simulink model "GateMate_SingleWire_TxRx_RGBW"  (R2025b)
settings: Solver=VariableStepAuto  StartTime=0.0  StopTime=simStopTime  RelTol=1e-3
libraries: ee_lib x17, simulink x9, fl_lib x9, nesl_utility x9
settings Model: Creator=Sneha Shree K  LastModifiedBy=Sneha Shree K

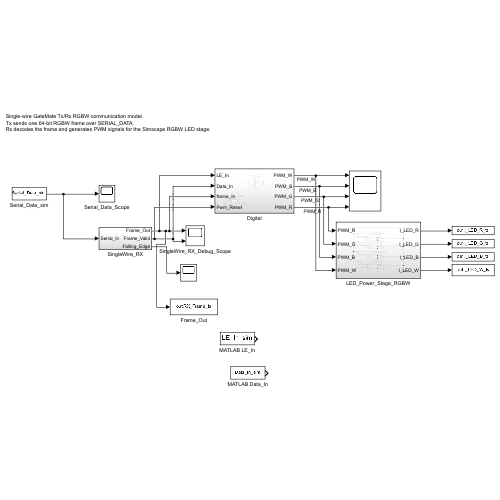
[thumbnail: Simulink's stored preview of the top-level diagram]
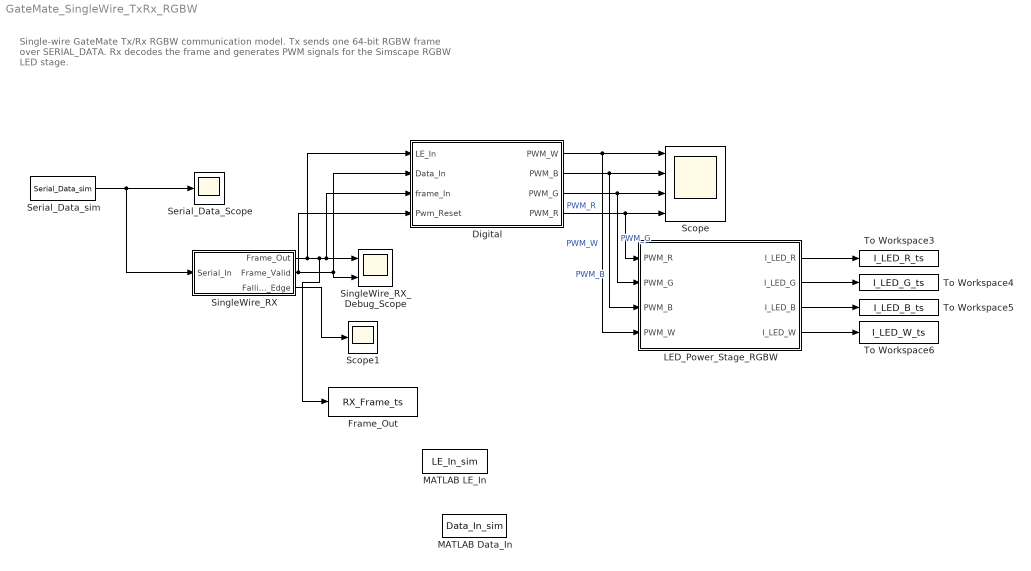
== system GateMate_SingleWire_TxRx_RGBW ==
  note: Single-wire GateMate Tx/Rx RGBW communication model.
      | Tx sends one 64-bit RGBW frame over SERIAL_DATA.
      | Rx decodes the frame and generates PWM signals for the Simscape RGBW LED stage.
  Digital : Subsystem
  Frame_Out : ToWorkspace  VariableName=RX_Frame_ts  SaveFormat=Timeseries  SampleTime=-1
  LED_Power_Stage_RGBW : Subsystem
  MATLAB Data_In : FromWorkspace  VariableName=Data_In_sim  Interpolate=off  OutputAfterFinalValue=Holding final value
  "MATLAB LE_In " : FromWorkspace  VariableName=LE_In_sim  Interpolate=off  OutputAfterFinalValue=Holding final value
  Scope : Scope  NumInputPorts=4
      settings: ActiveDisplayYMinimum=-0.41394567677319716  ActiveDisplayYMaximum=1.1355839256009383
  Scope1 : Scope
      settings: TimeSpan=0.22  ActiveDisplayYMinimum=-0.2  ActiveDisplayYMaximum=1.2  DataLoggingVariableName=ScopeData3
  Serial_Data_Scope : Scope
      settings: ActiveDisplayYMinimum=-0.12499999999999997  ActiveDisplayYMaximum=1.125
  "Serial_Data_sim " : FromWorkspace  VariableName=Serial_Data_sim
  SingleWire_RX : Subsystem
  SingleWire_RX_Debug_Scope : Scope  NumInputPorts=2
      settings: ActiveDisplayYMinimum=-1  ActiveDisplayYMaximum=1  DataLoggingVariableName=ScopeData2
  To Workspace3 : ToWorkspace  VariableName=I_LED_R_ts  SaveFormat=Timeseries  SampleTime=-1
  To Workspace4 : ToWorkspace  VariableName=I_LED_G_ts  SaveFormat=Timeseries  SampleTime=-1
  To Workspace5 : ToWorkspace  VariableName=I_LED_B_ts  SaveFormat=Timeseries  SampleTime=-1
  To Workspace6 : ToWorkspace  VariableName=I_LED_W_ts  SaveFormat=Timeseries  SampleTime=-1
  wires:
  Digital/1(PWM_W) -> LED_Power_Stage_RGBW/4(PWM_W), Scope/1  "PWM_W"
  Digital/2(PWM_B) -> LED_Power_Stage_RGBW/3(PWM_B), Scope/2  "PWM_B"
  Digital/3(PWM_G) -> LED_Power_Stage_RGBW/2(PWM_G), Scope/3  "PWM_G"
  Digital/4(PWM_R) -> LED_Power_Stage_RGBW/1(PWM_R), Scope/4  "PWM_R"
  LED_Power_Stage_RGBW/1(I_LED_R) -> To Workspace3/1
  LED_Power_Stage_RGBW/2(I_LED_G) -> To Workspace4/1
  LED_Power_Stage_RGBW/3(I_LED_B) -> To Workspace5/1
  LED_Power_Stage_RGBW/4(I_LED_W) -> To Workspace6/1
  "Serial_Data_sim "/1 -> SingleWire_RX/1(Serial_In), Serial_Data_Scope/1
  SingleWire_RX/1(Frame_Out) -> Digital/3(frame_In), SingleWire_RX_Debug_Scope/1, Frame_Out/1, Digital/1(LE_In)
  SingleWire_RX/2(Frame_Valid) -> Digital/4(Pwm_Reset), SingleWire_RX_Debug_Scope/2, Digital/2(Data_In)
  SingleWire_RX/3(Falling_Edge) -> Scope1/1

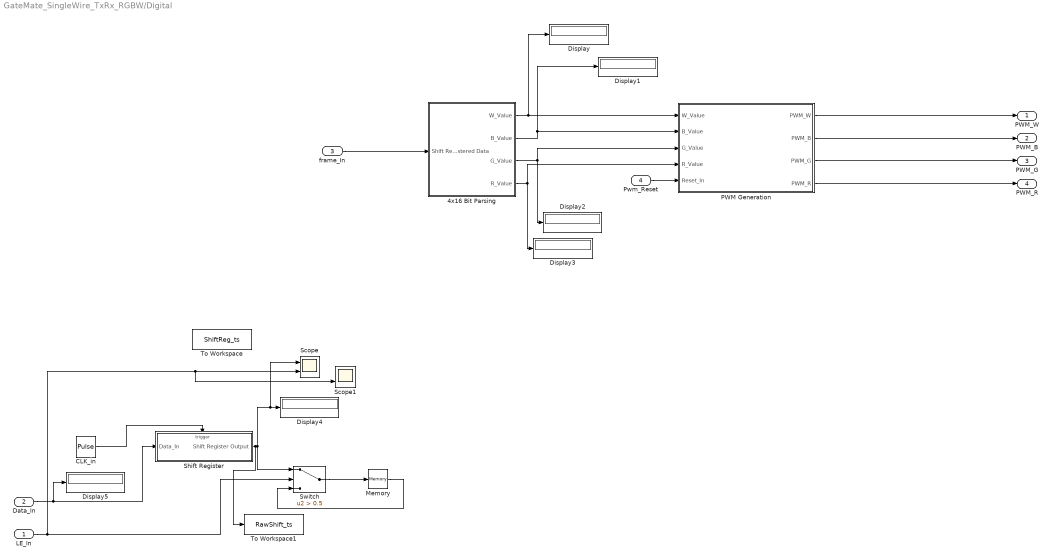
== system GateMate_SingleWire_TxRx_RGBW/Digital ==
  LE_In : Inport
  Data_In : Inport  Port=2
  frame_In : Inport  Port=3  OutDataTypeStr=uint64
  Pwm_Reset : Inport  Port=4  OutDataTypeStr=boolean
  4x16 Bit Parsing : Subsystem
  CLK_in : DiscretePulseGenerator  PulseType=Time based  Period=1e-3  PulseWidth=50  PhaseDelay=0.5e-3
  Display{,1..5} (6 alike) : Display
  Memory : Memory
  PWM Generation : Subsystem
  Scope : Scope  NumInputPorts=2
      settings: ActiveDisplayYMinimum=-0.12499999999999997  ActiveDisplayYMaximum=1.125  DataLoggingVariableName=ScopeData4
  Scope1 : Scope  NumInputPorts=2
      settings: ActiveDisplayYMinimum=-0.12499999999999997  ActiveDisplayYMaximum=1.125  DataLoggingVariableName=ScopeData5
  Shift Register : Subsystem  TreatAsAtomicUnit=on
  Switch : Switch  Criteria=u2 > Threshold  Threshold=0.5  SaturateOnIntegerOverflow=off  InputSameDT=off
  To Workspace : ToWorkspace  VariableName=ShiftReg_ts  SaveFormat=Timeseries  SampleTime=-1
  To Workspace1 : ToWorkspace  VariableName=RawShift_ts  SaveFormat=Timeseries  SampleTime=-1
  PWM_W : Outport
  PWM_B : Outport  Port=2
  PWM_G : Outport  Port=3
  PWM_R : Outport  Port=4
  wires:
  CLK_in/1 -> Shift Register/Trigger
  Data_In/1 -> Display5/1, Shift Register/1(Data_In)
  Switch/1 -> Memory/1
  Memory/1 -> Switch/3
  Shift Register/1(Shift Register Output) -> To Workspace1/1, Scope/1, Display4/1, Switch/1
  LE_In/1 -> Scope1/2, Scope/2, Switch/2
  4x16 Bit Parsing/1(W_Value) -> Display/1, PWM Generation/1(W_Value)
  4x16 Bit Parsing/2(B_Value) -> Display1/1, PWM Generation/2(B_Value)
  4x16 Bit Parsing/3(G_Value) -> Display2/1, PWM Generation/3(G_Value)
  4x16 Bit Parsing/4(R_Value) -> Display3/1, PWM Generation/4(R_Value)
  PWM Generation/1(PWM_W) -> PWM_W/1
  PWM Generation/2(PWM_B) -> PWM_B/1
  PWM Generation/3(PWM_G) -> PWM_G/1
  PWM Generation/4(PWM_R) -> PWM_R/1
  frame_In/1 -> 4x16 Bit Parsing/1(Shift Registered Data)
  Pwm_Reset/1 -> PWM Generation/5(Reset_In)

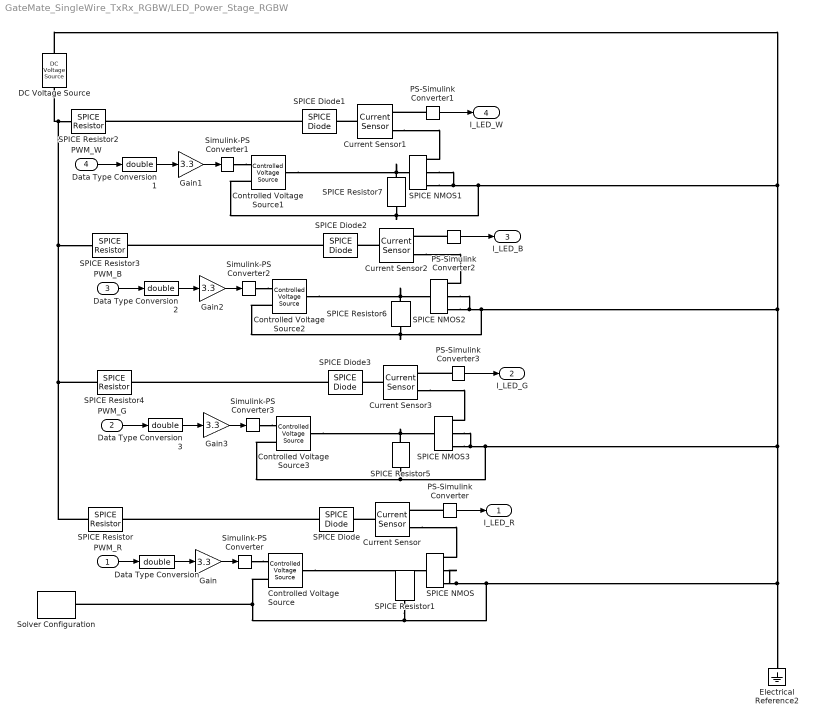
== system GateMate_SingleWire_TxRx_RGBW/LED_Power_Stage_RGBW ==
  PWM_R : Inport
  PWM_G : Inport  Port=2
  PWM_B : Inport  Port=3
  PWM_W : Inport  Port=4
  Controlled Voltage Source{,1..3} (4 alike) : fl_lib/Electrical/Electrical Sources/Controlled Voltage Source
  Current Sensor{,1..3} (4 alike) : fl_lib/Electrical/Electrical Sensors/Current Sensor
  DC Voltage Source : ee_lib/Additional Components/SPICE Sources/DC Voltage Source  DC=12 V
  Data Type Conversion{,1..3} (4 alike) : DataTypeConversion  OutDataTypeStr=double  SaturateOnIntegerOverflow=off  RndMeth=Floor
  Electrical Reference2 : fl_lib/Electrical/Electrical Elements/Electrical Reference
  Gain{,1..3} (4 alike) : Gain  Gain=3.3
  PS-Simulink Converter{,1..3} (4 alike) : nesl_utility/PS-Simulink Converter  PhysicalDomain=network_engine_domain  SubClassName=ps_output  LeftPortType=input  RightPortType=output  PseudoPeriodic=off  Frequencies=[]  VectorFormat=inherit  Unit=A  AffineConversion=off
  SPICE Diode{,1..3} (4 alike) : ee_lib/Additional Components/SPICE Semiconductors/SPICE Diode  AREA=1.0 m^2  SCALE=1  IS=1e-14 A/m^2  IKF=Inf A/m^2  ISR=0 A/m^2  N=1  NR=2  M=0.5  VJ=1 V  RS=0.01 Ohm*m^2  C_param=1  CJO=0 F/m^2  FC=0.5  TT=0 s  IC_given=1  V0=0 V  RevBrk=1  BV=Inf V  IBV=1e-10 A/m^2  IBVL=0 A/m^2  NBV=1  NBVL=1  T_param=1  XTI=3.0  EG=1.11 eV  TIKF=0 1/K  TRS1=0 1/K  TRS2=0 1/K^2  TBV1=0 1/K  TBV2=0 1/K^2  TFIXED=300.15 K  TMEAS=300.15 K  TOFFSET=0 K
      settings: InternalSimscapePortConfiguration="{\"Bottom\":[],\"Left\":[{\"id\":\"p\",\"label\":\"+\",\"type\":\"foundation.electrical.electrical\"}],\"Right\":[{\"id\":\"n\",\"label\":\"-\",\"type\":\"foundation.electrical.electrical\"}],\"Top\":[]}"
  SPICE NMOS{,1..3} (4 alike) : ee_lib/Additional Components/SPICE Semiconductors/SPICE NMOS  LEVEL=1  AREA=1.0  SCALE=1  LENGTH=1e-4 m  WIDTH=1e-4 m  AD=0 m^2  AS=0 m^2  PD=0 m  PS=0 m  NRD=0  NRS=0  RD=0.05 Ohm  RS=0.05 Ohm  RSH=0 Ohm  VTO=1.5 V  KP=1 A/V^2  GAMMA=0 V^(1/2)  PHI=0.6 V  LAMBDA=0 1/V  IS=1e-14 A  N=1  JS=0 A/m^2  DELTA=0  VMAX=0 m/s  NFS=0 1/cm^2  ETA=0  THETA=0 1/V  KAPPA=0.2  Ci_param=ee.enum.intrinsicCapacitance.none  Cov_param=ee.enum.includeCapacitance.no  CGSO=0 F/m  CGDO=0 F/m  CGBO=0 F/m  C_param=ee.enum.includeCapacitance.no  CBD=0 F  CBS=0 F  PB=0.8 V  CJ=0 F/m^2  MJ=0.5  CJSW=0 F/m  MJSW=0.5  FC=0.5  IC_given=ee.enum.initialCondition.no  ICVDS=0 V  ICVGS=0 V  ICVBS=0 V  TOX=1e-7 m  LD=0 m  U0=600 cm^2/(V*s)  NSUB=NaN 1/cm^3  TPG=1  NSS=NaN 1/cm^2  XJ=0 m  T_param=1  TFIXED=300.15 K  TMEAS=300.15 K  TOFFSET=0 K  UEXP=0  UCRIT=1e4 V/cm  NEFF=1  MTYPE=1
      settings: InternalSimscapePortConfiguration="{\"Bottom\":[],\"Left\":[{\"id\":\"gx\",\"label\":\"\",\"type\":\"foundation.electrical.electrical\"}],\"Right\":[{\"id\":\"dx\",\"label\":\"\",\"type\":\"foundation.electrical.electrical\"},{\"id\":\"bx\",\"label\":\"\",\"type\":\"foundation.electrical.electrical\"},{\"id\":\"sx\",\"label\":\"\",\"type\":\"foundation.electrical.electrical\"}],\"Top\":[]}"
  SPICE Resistor{,2..4} (4 alike) : ee_lib/Additional Components/SPICE Passives/SPICE Resistor  SCALE=1.0  R_param=1  R=510 Ohm  RSH=0 Ohm  LENGTH=1e-6 m  WIDTH=1e-6 m  NARROW=0 m  T_param=1  TC1=0 1/K  TC2=0 1/K^2  TOFFSET=0 K  TFIXED=300.15 K  TMEAS=300.15 K
      settings: InternalSimscapePortConfiguration="{\"Bottom\":[],\"Left\":[{\"id\":\"p\",\"label\":\"\",\"type\":\"foundation.electrical.electrical\"}],\"Right\":[{\"id\":\"n\",\"label\":\"\",\"type\":\"foundation.electrical.electrical\"}],\"Top\":[]}"
  SPICE Resistor{1,5..7} (4 alike) : ee_lib/Additional Components/SPICE Passives/SPICE Resistor  SCALE=1.0  R_param=1  R=100 kOhm  RSH=0 Ohm  LENGTH=1e-6 m  WIDTH=1e-6 m  NARROW=0 m  T_param=1  TC1=0 1/K  TC2=0 1/K^2  TOFFSET=0 K  TFIXED=300.15 K  TMEAS=300.15 K
      settings: InternalSimscapePortConfiguration="{\"Bottom\":[],\"Left\":[{\"id\":\"p\",\"label\":\"\",\"type\":\"foundation.electrical.electrical\"}],\"Right\":[{\"id\":\"n\",\"label\":\"\",\"type\":\"foundation.electrical.electrical\"}],\"Top\":[]}"
  Simulink-PS Converter{,1..3} (4 alike) : nesl_utility/Simulink-PS Converter  PhysicalDomain=network_engine_domain  SubClassName=ps_input  LeftPortType=input  RightPortType=output  PseudoPeriodic=off  Frequencies=[]  NoiseDistribution=none  NoiseParameters=[]  Unit=V  AffineConversion=off  FilteringAndDerivatives=provide  SimscapeFilterOrder=1  InputFilterTimeConstant=0.001  UdotUserProvided=0
  Solver Configuration : nesl_utility/Solver Configuration  PhysicalDomain=network_engine_domain  SubClassName=solver  LeftPortType=input  RightPortType=generic  Tones=[]  Harmonics=[]  SimulateNoise=off  Profile=off  UseLocalSampling=off  EnableSwitchedLinearOptims=on  FrequencyDomain=off  UseCCode=off  RelTol=0.001  AbsTol=0.001  MinStep=1e-09  ToWorkspace=off  RevertToSquareIcSolve=off  NumHomotopyIterations=100  PhasorMode=off  PhasorModeNumHarmonics=1  ConsistencySolver=NEWTON_XTOL_AFTER_FTOL  IndexReductionMethod=DerivativeReplacement  DoDC=off  ResidualTolerance=1e-09  ConsistencyTolSource=GLOBAL  ConsistencyAbsTol=0.001  ConsistencyRelTol=0.001  ConsistencyTolFactor=0.001  UseLocalSolver=off  LocalSolverChoice=NE_BACKWARD_EULER_ADVANCER  ResolveIndetEquations=on  FunctionEvalNumThread=1  LocalSolverSampleTime=0.001  DoFixedCost=off  MaxNonlinIter=3  MaxModeIter=2  ComputeImpulses=off  ImpulseIterations=2  LinearAlgebra=auto  LinearAlgebraNumThread=0  EquationFormulation=NE_TIME_EF  DelaysMemoryBudget=1024  AutomaticFiltering=on  FilteringTimeConstant=0.001  PartitionStorageMethod=AS_NEEDED  PartitionMemoryBudget=1024  PartitionMethod=ROBUST  MultibodyUseLocalSolver=off  MultibodyLocalSolverChoice=ODE1  MultibodyLocalSolverSampleTime=0.001
  I_LED_R : Outport  VectorParamsAs1DForOutWhenUnconnected=off
  I_LED_G : Outport  Port=2  VectorParamsAs1DForOutWhenUnconnected=off
  I_LED_B : Outport  Port=3  VectorParamsAs1DForOutWhenUnconnected=off
  I_LED_W : Outport  Port=4  VectorParamsAs1DForOutWhenUnconnected=off
  wires:
  Gain/1 -> Simulink-PS Converter/1
  PS-Simulink Converter/1 -> I_LED_R/1
  PWM_R/1 -> Data Type Conversion/1
  Data Type Conversion/1 -> Gain/1
  Data Type Conversion1/1 -> Gain1/1
  Gain1/1 -> Simulink-PS Converter1/1
  PWM_W/1 -> Data Type Conversion1/1
  PS-Simulink Converter1/1 -> I_LED_W/1
  Data Type Conversion2/1 -> Gain2/1
  Gain2/1 -> Simulink-PS Converter2/1
  PWM_B/1 -> Data Type Conversion2/1
  PS-Simulink Converter2/1 -> I_LED_B/1
  Data Type Conversion3/1 -> Gain3/1
  Gain3/1 -> Simulink-PS Converter3/1
  PWM_G/1 -> Data Type Conversion3/1
  PS-Simulink Converter3/1 -> I_LED_G/1
  connections:
  SPICE Diode/LConn1 -- SPICE Resistor/RConn1
  Current Sensor/LConn1 -- SPICE Diode/RConn1
  Current Sensor/RConn2 -- SPICE NMOS/RConn1
  Controlled Voltage Source/LConn1 -- SPICE NMOS/LConn1
  Simulink-PS Converter/RConn1 -- Controlled Voltage Source/RConn1
  PS-Simulink Converter/LConn1 -- Current Sensor/RConn1
  SPICE Diode1/LConn1 -- SPICE Resistor2/RConn1
  Controlled Voltage Source1/LConn1 -- SPICE Resistor7/LConn1 -- SPICE NMOS1/LConn1
  Current Sensor1/RConn2 -- SPICE NMOS1/RConn1
  PS-Simulink Converter1/LConn1 -- Current Sensor1/RConn1
  Current Sensor1/LConn1 -- SPICE Diode1/RConn1
  Simulink-PS Converter1/RConn1 -- Controlled Voltage Source1/RConn1
  SPICE Diode2/LConn1 -- SPICE Resistor3/RConn1
  Controlled Voltage Source2/LConn1 -- SPICE Resistor6/LConn1 -- SPICE NMOS2/LConn1
  Current Sensor2/RConn2 -- SPICE NMOS2/RConn1
  PS-Simulink Converter2/LConn1 -- Current Sensor2/RConn1
  Current Sensor2/LConn1 -- SPICE Diode2/RConn1
  Simulink-PS Converter2/RConn1 -- Controlled Voltage Source2/RConn1
  SPICE Resistor/LConn1 -- SPICE Resistor4/LConn1 -- SPICE Resistor3/LConn1 -- DC Voltage Source/LConn1 -- SPICE Resistor2/LConn1
  SPICE Diode3/LConn1 -- SPICE Resistor4/RConn1
  Controlled Voltage Source3/LConn1 -- SPICE Resistor5/LConn1 -- SPICE NMOS3/LConn1
  Current Sensor3/RConn2 -- SPICE NMOS3/RConn1
  PS-Simulink Converter3/LConn1 -- Current Sensor3/RConn1
  Current Sensor3/LConn1 -- SPICE Diode3/RConn1
  Simulink-PS Converter3/RConn1 -- Controlled Voltage Source3/RConn1
  Controlled Voltage Source/RConn2 -- SPICE NMOS/RConn2 -- SPICE NMOS/RConn3 -- SPICE Resistor5/RConn1 -- Controlled Voltage Source3/RConn2 -- SPICE NMOS3/RConn2 -- SPICE NMOS3/RConn3 -- SPICE Resistor7/RConn1 -- Controlled Voltage Source1/RConn2 -- SPICE NMOS1/RConn2 -- SPICE NMOS1/RConn3 -- DC Voltage Source/RConn1 -- SPICE Resistor6/RConn1 -- Controlled Voltage Source2/RConn2 -- SPICE NMOS2/RConn2 -- SPICE NMOS2/RConn3 -- Electrical Reference2/LConn1 -- SPICE Resistor1/RConn1 -- Solver Configuration/RConn1

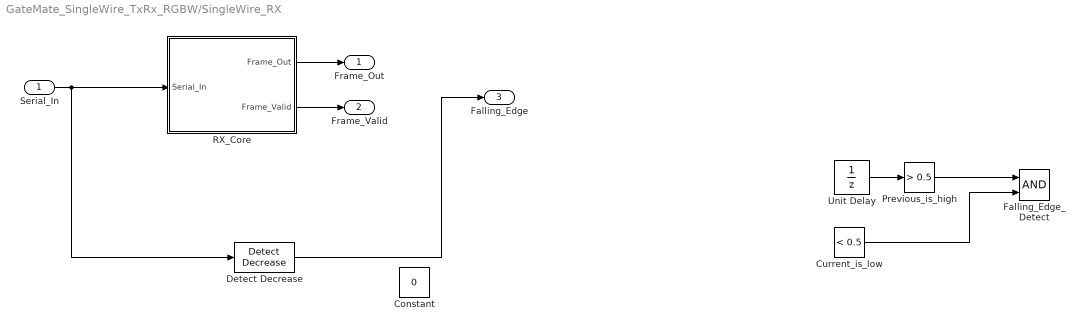
== system GateMate_SingleWire_TxRx_RGBW/SingleWire_RX ==
  Serial_In : Inport
  Constant : Constant  Value=0
  Current_is_low : simulink/Logic and Bit Operations/Compare To Constant  relop=<  const=0.5  OutDataTypeStr=boolean
  Detect Decrease : simulink/Logic and Bit Operations/Detect Decrease  vinit=0.0  OutDataTypeStr=boolean
  Falling_Edge_Detect : Logic  AllPortsSameDT=off  OutDataTypeStr=boolean
  Previous_is_high : simulink/Logic and Bit Operations/Compare To Constant  relop=>  const=0.5  OutDataTypeStr=boolean
  RX_Core : MATLAB Function  TreatAsAtomicUnit=on
  Unit Delay : UnitDelay  InitialCondition=1  HasFrameUpgradeWarning=on
  Frame_Out : Outport  OutDataTypeStr=uint64
  Frame_Valid : Outport  Port=2  OutDataTypeStr=boolean
  Falling_Edge : Outport  Port=3
  wires:
  Serial_In/1 -> RX_Core/1(Serial_In), Detect Decrease/1
  Detect Decrease/1 -> Falling_Edge/1
  ? -> Current_is_low/1, Unit Delay/1
  Unit Delay/1 -> Previous_is_high/1
  Previous_is_high/1 -> Falling_Edge_Detect/1
  Current_is_low/1 -> Falling_Edge_Detect/2
  RX_Core/1(Frame_Out) -> Frame_Out/1
  RX_Core/2(Frame_Valid) -> Frame_Valid/1

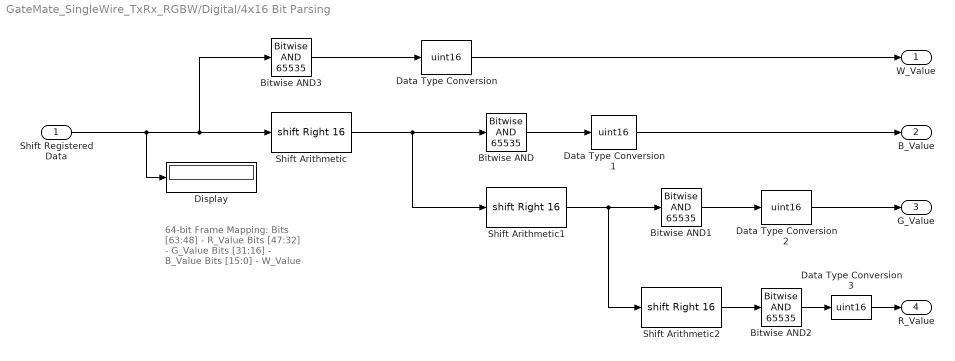
== system GateMate_SingleWire_TxRx_RGBW/Digital/4x16 Bit Parsing ==
  note: 64-bit Frame Mapping:
      |
      | Bits [63:48] - R_Value
      | Bits [47:32] - G_Value
      | Bits [31:16] - B_Value
      | Bits [15:0] - W_Value
  Shift Registered Data : Inport  OutDataTypeStr=uint64
  Bitwise AND{,1..3} (4 alike) : simulink/Logic and Bit Operations/Bitwise Operator  logicop=AND  UseBitMask=on  BitMask=65535  BitMaskRealWorld=Stored Integer
      settings: LibrarySourceBlock=|
      | simulink/Quick Insert/Logic and Bit
      | Operations/Bitwise AND
  Data Type Conversion{,1..3} (4 alike) : DataTypeConversion  OutDataTypeStr=uint16  SaturateOnIntegerOverflow=off  RndMeth=Floor
  Display : Display
  Shift Arithmetic : ArithShift  BitShiftNumber=16  BitShiftDirection=Right
  Shift Arithmetic1 : ArithShift  BitShiftNumber=16  BitShiftDirection=Right
  Shift Arithmetic2 : ArithShift  BitShiftNumber=16  BitShiftDirection=Right
  W_Value : Outport
  B_Value : Outport  Port=2
  G_Value : Outport  Port=3
  R_Value : Outport  Port=4
  wires:
  Shift Arithmetic/1 -> Shift Arithmetic1/1, Bitwise AND/1
  Shift Registered Data/1 -> Display/1, Shift Arithmetic/1, Bitwise AND3/1
  Shift Arithmetic1/1 -> Shift Arithmetic2/1, Bitwise AND1/1
  Shift Arithmetic2/1 -> Bitwise AND2/1
  Bitwise AND3/1 -> Data Type Conversion/1
  Bitwise AND/1 -> Data Type Conversion1/1
  Bitwise AND1/1 -> Data Type Conversion2/1
  Bitwise AND2/1 -> Data Type Conversion3/1
  Data Type Conversion/1 -> W_Value/1
  Data Type Conversion1/1 -> B_Value/1
  Data Type Conversion2/1 -> G_Value/1
  Data Type Conversion3/1 -> R_Value/1

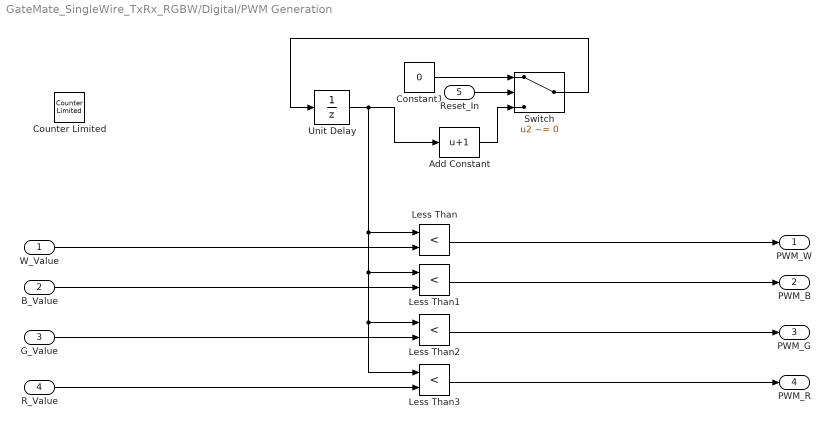
== system GateMate_SingleWire_TxRx_RGBW/Digital/PWM Generation ==
  W_Value : Inport
  B_Value : Inport  Port=2
  G_Value : Inport  Port=3
  R_Value : Inport  Port=4
  Reset_In : Inport  Port=5
  Add Constant : Bias  Bias=1  SaturateOnIntegerOverflow=off
  Constant1 : Constant  Value=0  OutDataTypeStr=uint16
  Counter Limited : simulink/Sources/Counter Limited  uplimit=65535  tsamp=1e-6
  Less Than{,1..3} (4 alike) : RelationalOperator  Operator=<  OutDataTypeStr=boolean  RndMeth=Simplest  InputSameDT=off
  Switch : Switch  Criteria=u2 ~= 0  SaturateOnIntegerOverflow=off  InputSameDT=off
  Unit Delay : UnitDelay  SampleTime=1e-6  HasFrameUpgradeWarning=on
  PWM_W : Outport
  PWM_B : Outport  Port=2
  PWM_G : Outport  Port=3
  PWM_R : Outport  Port=4
  wires:
  W_Value/1 -> Less Than/2
  Less Than/1 -> PWM_W/1
  B_Value/1 -> Less Than1/2
  G_Value/1 -> Less Than2/2
  Less Than1/1 -> PWM_B/1
  Less Than2/1 -> PWM_G/1
  Less Than3/1 -> PWM_R/1
  R_Value/1 -> Less Than3/2
  Constant1/1 -> Switch/1
  Reset_In/1 -> Switch/2
  Add Constant/1 -> Switch/3
  Unit Delay/1 -> Less Than2/1, Less Than3/1, Less Than1/1, Less Than/1, Add Constant/1
  Switch/1 -> Unit Delay/1

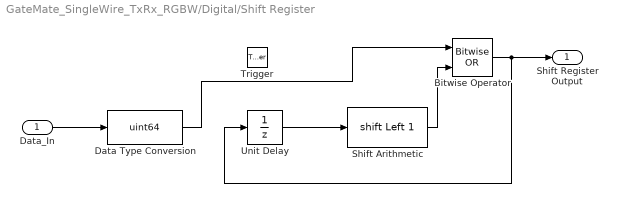
== system GateMate_SingleWire_TxRx_RGBW/Digital/Shift Register ==
  Data_In : Inport
  Trigger : TriggerPort  VariantControl=(inherit)
  Bitwise Operator : simulink/Logic and Bit Operations/Bitwise Operator  logicop=OR  UseBitMask=off  NumInputPorts=2  BitMask=bin2dec('11011001')  BitMaskRealWorld=Stored Integer
  Data Type Conversion : DataTypeConversion  OutDataTypeStr=uint64  SaturateOnIntegerOverflow=off  RndMeth=Floor
  Shift Arithmetic : ArithShift  BitShiftNumber=1  BitShiftDirection=Left
  Unit Delay : UnitDelay  SampleTime=-1  HasFrameUpgradeWarning=on
  Shift Register Output : Outport  OutDataTypeStr=uint64
  wires:
  Data_In/1 -> Data Type Conversion/1
  Unit Delay/1 -> Shift Arithmetic/1
  Shift Arithmetic/1 -> Bitwise Operator/2
  Data Type Conversion/1 -> Bitwise Operator/1
  Bitwise Operator/1 -> Shift Register Output/1, Unit Delay/1

== matlab function GateMate_SingleWire_TxRx_RGBW/SingleWire_RX/RX_Core ==
  settings: updateMethod=DISCRETE  sampleTime=0.00025
  data: Serial_In input; Frame_Out output; Frame_Valid output
function [Frame_Out, Frame_Valid] = RX_Core(Serial_In)
% Simple single-wire 64-bit RGBW receiver
%
% Ts   = 0.25 ms
% Tbit = 1 ms
% 4 samples per bit
%
% Frame:
% Idle HIGH
% Start bit LOW
% 64 data bits, MSB first
% Stop bit HIGH

persistent active
persistent sample_count
persistent bit_count
persistent shift_reg
persistent latched_frame
persistent previous_value

if isempty(active)
    active         = false;
    sample_count   = uint16(0);
    bit_count      = uint16(0);
    shift_reg      = uint64(0);
    latched_frame  = uint64(0);
    previous_value = 1;
end

%% Default outputs

% IMPORTANT:
% Output only the last COMPLETE frame.
% Do not output the partially received shift register.
Frame_Out   = latched_frame;
Frame_Valid = false;

%% IDLE STATE

if ~active

    % Detect falling edge:
    % Idle HIGH -> Start bit LOW
    if (previous_value > 0.5) && (Serial_In < 0.5)

        active       = true;
        sample_count = uint16(0);
        bit_count    = uint16(0);
        shift_reg    = uint64(0);

    end

%% RECEIVE STATE

else

    sample_count = sample_count + 1;

    % Sample approximately at the centre of every data bit.
    %
    % Start bit occupies approximately samples 0...3.
    % First data-bit sample occurs at sample 6.
    % Then sample every 4 samples.

    if sample_count >= 6 && ...
       mod(double(sample_count - 6), 4) == 0 && ...
       bit_count < 64

        % Shift previous bits left
        shift_reg = bitshift(shift_reg, 1);

        % Insert new bit into LSB
        if Serial_In > 0.5
            shift_reg = bitor(shift_reg, uint64(1));
        end

        bit_count = bit_count + 1;
    end

    %% Complete frame received

    if bit_count == 64

        % Latch the COMPLETE frame
        latched_frame = shift_reg;

        % Update output
        Frame_Out = latched_frame;

        % One-sample valid pulse
        Frame_Valid = true;

        % Return receiver to idle
        active       = false;
        sample_count = uint16(0);
        bit_count    = uint16(0);

    end
end

previous_value = Serial_In;

end
